simulink model "openloop_SPWM_v2_2020a"  (R2020a)
settings: Solver=ode23tb  StartTime=0.0  StopTime=2  MaxStep=1e-4  RelTol=1e-7
values from neighbouring files (symbols this model uses):
  J = 0.02    [parameter.mat]
  Lm = 0.3197    [parameter.mat]
  Lr = 0.33003    [parameter.mat]
  Ls = 0.33003    [parameter.mat]
  np = 2    [parameter.mat]
  Rr = 2.178    [parameter.mat]
  Rs = 2.804    [parameter.mat]
  Tr = 0.15152892562    [parameter.mat]
libraries: powerlib x9, powerlib_meascontrol x4
settings Model: Creator=Yeblue  LastModifiedBy=EVA
settings DebuggingCC: SFMachineParentedDataDiag=error

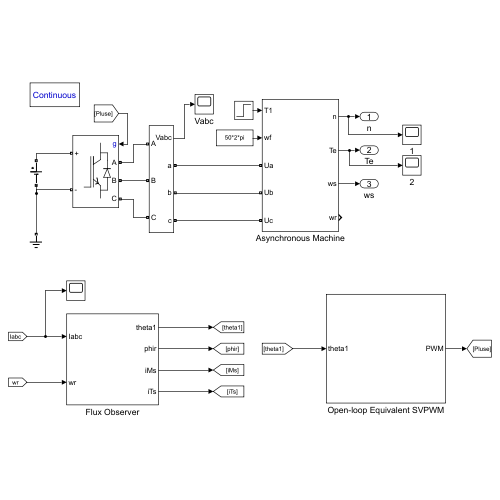
[thumbnail: Simulink's stored preview of the top-level diagram]
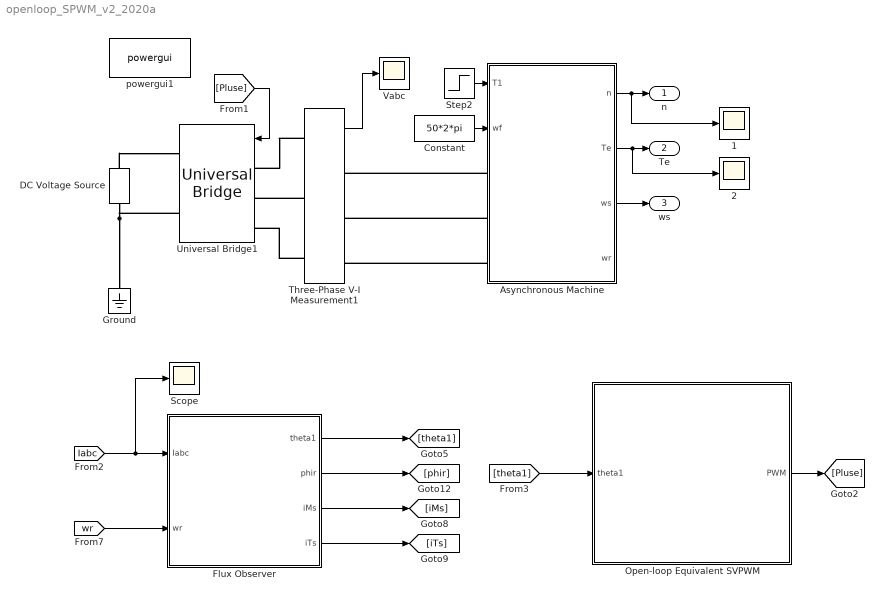
== system openloop_SPWM_v2_2020a ==
  1 : Scope
  2 : Scope
  Asynchronous Machine : Subsystem
  Constant : Constant  Value=50*2*pi
  DC Voltage Source : powerlib/Electrical Sources/DC Voltage Source  Amplitude=380*sqrt(2)/0.5  Measurements=None
  Flux Observer : Subsystem
  Ground : powerlib/Elements/Ground  LConnTagsString=a
  Open-loop Equivalent SVPWM : Subsystem
  Scope : Scope
  Step2 : Step  After=5  SampleTime=0
  Three-Phase V-I Measurement1 : powerlib/Measurements/Three-Phase V-I Measurement  VoltageMeasurement=phase-to-phase  SetLabelV=off  LabelV=Vabc  Vpu=off  VpuLL=off  CurrentMeasurement=no  SetLabelI=off  LabelI=Iabc  Ipu=off  Pbase=100e6  Vbase=500e3  OutputType=Complex  PhasorSimulation=off  PSBequivalent=0
  Universal Bridge1 : powerlib/Power Electronics/Universal Bridge  Arms=3  SnubberResistance=1e5  SnubberCapacitance=inf  Device=IGBT / Diodes  Ron=1e-3  Lon=0  ForwardVoltages="[  0  0  ]"  ForwardVoltage=0  GTOparameters=[ 10e-6 , 20e-6 ]  IGBTparameters=[ 1e-6 , 2e-6 ]  Measurements=None  Measurements_2=None  converterType=Rectifier
  Vabc : Scope
  powergui1 : powerlib/powergui  Priority=1  SimulationMode=Continuous  SampleTime=50e-6  frequency=60  Iterations=50  frequencyindice=0  Pbase=100e6  ErrMax=1e-4  UnitsV=kV  UnitsW=MW  buscounter=0  FunctionMessages=off  echomessages=off  EnableUseOfTLC=off  CurrentSourceSwitches=off  DisableSnubberDevices=off  DisableRonSwitches=off  DisableVfSwitches=off  DisplayEquations=off  AutomaticDiscreteSolvers=off  SolverType=Tustin/Backward Euler (TBE)  Interpol=off  ExternalGateDelay=off  methode=off  Ts=100  x0status=blocks  SPID=on  SwTol=0  HookPort=off  NonlinearTolerance=1e-4  nMaxIteration=100  ContinueOnMaxIteration=off  RestoreLinks=warning  ResistiveCurrentMeasurement=off  Frange=[0:2:500]  Ylog=off  Xlog=on  ShowGrid=off  save=off  variable=ZData  structure=Uab  ZoomFFT=off  StartTime=1.0  cycles=1  DisplayStyle=1  fundamental=50  FreqAxis=on  MaxFrequency=1000  frequencyindicesteady=1  RmsSteady=1  display=off
  n : Outport
  Te : Outport  Port=2
  ws : Outport  Port=3
  wires:
  Asynchronous Machine/2(Te) -> 2/1, Te/1
  Constant/1 -> Asynchronous Machine/2(wf)
  Step2/1 -> Asynchronous Machine/1(T1)
  Flux Observer/2(phir) -> [phir]
  [wr] -> Flux Observer/2(wr)
  [Pluse] -> Universal Bridge1/1
  Flux Observer/4(iTs) -> [iTs]
  Three-Phase V-I Measurement1/1 -> Vabc/1
  Flux Observer/3(iMs) -> [iMs]
  Flux Observer/1(theta1) -> [theta1]
  Asynchronous Machine/1(n) -> n/1, 1/1
  Asynchronous Machine/3(ws) -> ws/1
  [Iabc] -> Scope/1, Flux Observer/1(Iabc)
  Open-loop Equivalent SVPWM/1(PWM) -> [Pluse]
  [theta1] -> Open-loop Equivalent SVPWM/1(theta1)
  connections:
  Universal Bridge1/RConn2 -- Ground/LConn1 -- DC Voltage Source/LConn1
  Asynchronous Machine/LConn2 -- Three-Phase V-I Measurement1/RConn2
  Asynchronous Machine/LConn1 -- Three-Phase V-I Measurement1/RConn1
  Asynchronous Machine/LConn3 -- Three-Phase V-I Measurement1/RConn3
  Three-Phase V-I Measurement1/LConn3 -- Universal Bridge1/LConn3
  Three-Phase V-I Measurement1/LConn1 -- Universal Bridge1/LConn1
  Three-Phase V-I Measurement1/LConn2 -- Universal Bridge1/LConn2
  DC Voltage Source/RConn1 -- Universal Bridge1/RConn1

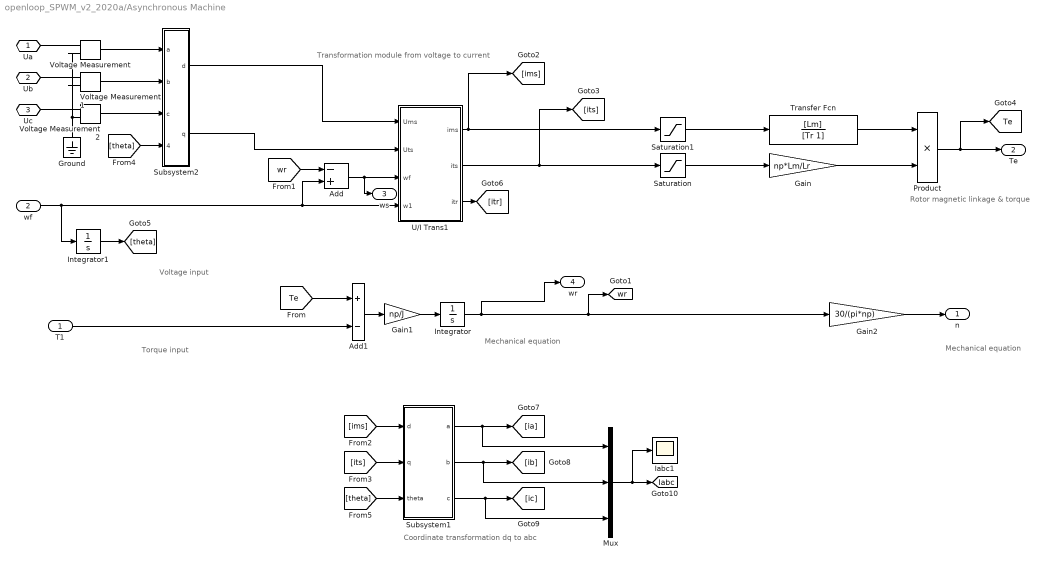
== system openloop_SPWM_v2_2020a/Asynchronous Machine ==
  note: Torque input
  note: Voltage input
  note: Rotor magnetic linkage & torque
  note: Transformation module from voltage to current
  note: Mechanical equation
  note: Coordinate transformation dq to abc
  note: Mechanical equation
  T1 : Inport
  wf : Inport  Port=2
  Add : Sum  Inputs=-+
  Add1 : Sum  Inputs=+-
  Gain : Gain  Gain=np*Lm/Lr
  Gain1 : Gain  Gain=np/J
  Gain2 : Gain  Gain=30/(pi*np)
  Ground : powerlib/Elements/Ground  LConnTagsString=a
  Iabc1 : Scope
  Integrator : Integrator
  Integrator1 : Integrator
  Mux : Mux  Inputs=3
  Product : Product
  Saturation : Saturate  UpperLimit=50  LowerLimit=-50
  Saturation1 : Saturate  UpperLimit=50  LowerLimit=-50
  Subsystem1 : Subsystem
  Subsystem2 : Subsystem
  Transfer Fcn : TransferFcn  Numerator=[Lm]  Denominator=[Tr 1]
  U/I Trans1 : Subsystem
  Voltage Measurement : powerlib/Measurements/Voltage Measurement  PhasorSimulation=off  OutputType=Complex  PSBequivalent=0
  Voltage Measurement1 : powerlib/Measurements/Voltage Measurement  PhasorSimulation=off  OutputType=Complex  PSBequivalent=0
  Voltage Measurement2 : powerlib/Measurements/Voltage Measurement  PhasorSimulation=off  OutputType=Complex  PSBequivalent=0
  Ua : PMIOPort  Side=Left
  Ub : PMIOPort  Port=2  Side=Left
  Uc : PMIOPort  Port=3  Side=Left
  n : Outport
  Te : Outport  Port=2
  ws : Outport  Port=3
  wr : Outport  Port=4
  tag scope: Iabc=global, Te=global, wr=global
  wires:
  Subsystem1/3(c) -> Mux/3, [ic]
  wf/1 -> Integrator1/1, U/I Trans1/4(w1), Add/2
  Product/1 -> Te/1, [Te]
  U/I Trans1/2(its) -> Saturation/1, [its]
  Voltage Measurement2/1 -> Subsystem2/3(c)
  [theta] -> Subsystem2/4(theta)
  Gain2/1 -> n/1
  Add/1 -> ws/1, U/I Trans1/3(wf)
  U/I Trans1/1(ims) -> Saturation1/1, [ims]
  Add1/1 -> Gain1/1
  [theta] -> Subsystem1/3(theta)
  Voltage Measurement1/1 -> Subsystem2/2(b)
  Subsystem2/1(d) -> U/I Trans1/1(Ums)
  [its] -> Subsystem1/2(q)
  Voltage Measurement/1 -> Subsystem2/1(a)
  T1/1 -> Add1/2
  U/I Trans1/3(itr) -> [itr]
  [ims] -> Subsystem1/1(d)
  Integrator1/1 -> [theta]
  Integrator/1 -> [wr], Gain2/1, wr/1
  [wr] -> Add/1
  Gain1/1 -> Integrator/1
  Gain/1 -> Product/2
  Subsystem2/2(q) -> U/I Trans1/2(Uts)
  [Te] -> Add1/1
  Subsystem1/1(a) -> Mux/1, [ia]
  Subsystem1/2(b) -> Mux/2, [ib]
  Transfer Fcn/1 -> Product/1
  Mux/1 -> Iabc1/1, [Iabc]
  Saturation/1 -> Gain/1
  Saturation1/1 -> Transfer Fcn/1
  connections:
  Ground/LConn1 -- Voltage Measurement1/LConn2 -- Voltage Measurement/LConn2 -- Voltage Measurement2/LConn2
  Uc/RConn1 -- Voltage Measurement2/LConn1
  Ub/RConn1 -- Voltage Measurement1/LConn1
  Ua/RConn1 -- Voltage Measurement/LConn1

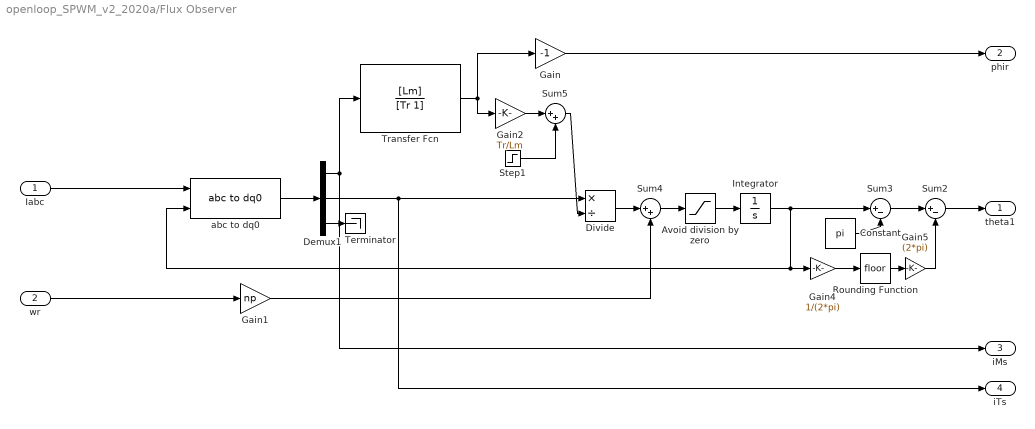
== system openloop_SPWM_v2_2020a/Flux Observer ==
  Iabc : Inport
  wr : Inport  Port=2
  Avoid division by zero : Saturate  UpperLimit=1e6  LowerLimit=1e-6
  Constant : Constant  Value=pi
  Demux1 : Demux  Outputs=3
  Divide : Product  Inputs=*/
  Gain : Gain  Gain=-1
  Gain1 : Gain  Gain=np
  Gain2 : Gain  Gain=Tr/Lm
  Gain4 : Gain  Gain=1/(2*pi)
  Gain5 : Gain  Gain=(2*pi)
  Integrator : Integrator  InitialCondition=10.00001
  Rounding Function : Rounding
  Step1 : Step  Time=0.01  Before=1000  After=0  SampleTime=0
  Sum2 : Sum  Inputs=|+-
  Sum3 : Sum  Inputs=|+-
  Sum4 : Sum  Inputs=|++
  Sum5 : Sum  Inputs=|++
  Terminator : Terminator
  Transfer Fcn : TransferFcn  Numerator=[Lm]  Denominator=[Tr 1]
  abc to dq0 : powerlib_meascontrol/Transformations/abc to dq0  Alignment=90 degrees behind phase A axis
  theta1 : Outport  VectorParamsAs1DForOutWhenUnconnected=off
  phir : Outport  Port=2  VectorParamsAs1DForOutWhenUnconnected=off
  iMs : Outport  Port=3  VectorParamsAs1DForOutWhenUnconnected=off
  iTs : Outport  Port=4  VectorParamsAs1DForOutWhenUnconnected=off
  wires:
  Divide/1 -> Sum4/1
  Step1/1 -> Sum5/2
  Sum5/1 -> Divide/2
  wr/1 -> Gain1/1
  Gain2/1 -> Sum5/1
  abc to dq0/1 -> Demux1/1
  Transfer Fcn/1 -> Gain/1, Gain2/1
  Iabc/1 -> abc to dq0/1
  Demux1/3 -> Terminator/1
  Demux1/1 -> iMs/1, Transfer Fcn/1
  Demux1/2 -> iTs/1, Divide/1
  Sum3/1 -> Sum2/1
  Sum2/1 -> theta1/1
  Constant/1 -> Sum3/2
  Rounding Function/1 -> Gain5/1
  Gain5/1 -> Sum2/2
  Gain4/1 -> Rounding Function/1
  Gain1/1 -> Sum4/2
  Gain/1 -> phir/1
  Sum4/1 -> Avoid division by zero/1
  Integrator/1 -> Sum3/1, Gain4/1, abc to dq0/2
  Avoid division by zero/1 -> Integrator/1

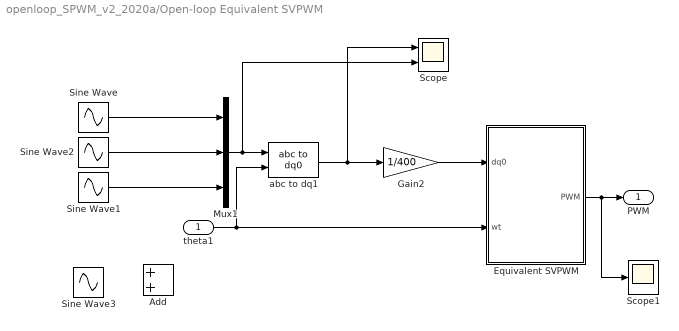
== system openloop_SPWM_v2_2020a/Open-loop Equivalent SVPWM ==
  theta1 : Inport
  Add : Sum
  Equivalent SVPWM : Subsystem
  Gain2 : Gain  Gain=1/400
  Mux1 : Mux  Inputs=3
  Scope : Scope  NumInputPorts=2
  Scope1 : Scope
  Sine Wave : Sin  Amplitude=380  Frequency=314.16  SampleTime=0
  Sine Wave1 : Sin  Amplitude=380  Frequency=314.16  Phase=2.0944  SampleTime=0
  Sine Wave2 : Sin  Amplitude=380  Frequency=314.16  Phase=4.1888  SampleTime=0
  Sine Wave3 : Sin  Amplitude=63.3333  Frequency=942.48  SampleTime=0
  abc to dq1 : powerlib_meascontrol/Transformations/abc to dq0  Alignment=90 degrees behind phase A axis
  PWM : Outport  VectorParamsAs1DForOutWhenUnconnected=off
  wires:
  theta1/1 -> Equivalent SVPWM/2(wt), abc to dq1/2
  Gain2/1 -> Equivalent SVPWM/1(dq0)
  Equivalent SVPWM/1(PWM) -> Scope1/1, PWM/1
  Sine Wave2/1 -> Mux1/2
  Sine Wave/1 -> Mux1/1
  Mux1/1 -> Scope/2, abc to dq1/1
  abc to dq1/1 -> Scope/1, Gain2/1
  Sine Wave1/1 -> Mux1/3

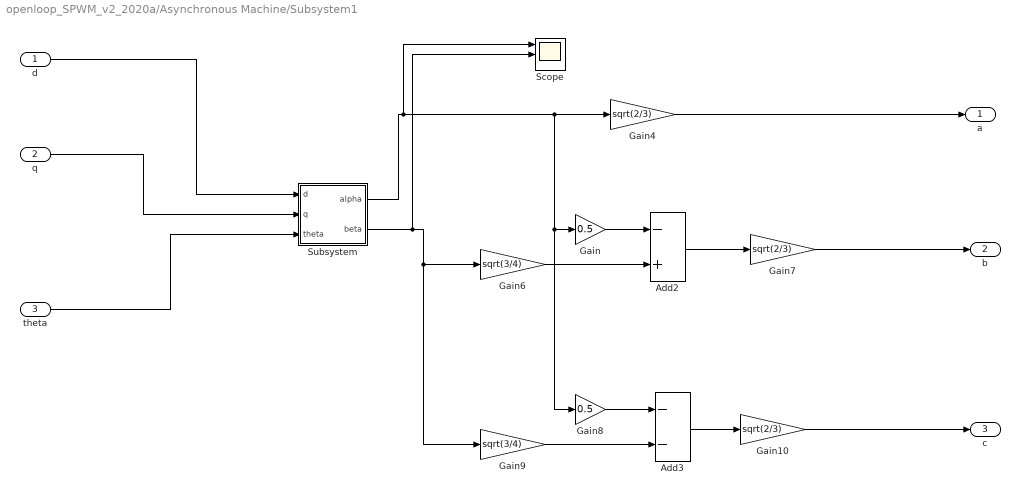
== system openloop_SPWM_v2_2020a/Asynchronous Machine/Subsystem1 ==
  d : Inport
  q : Inport  Port=2
  theta : Inport  Port=3
  Add2 : Sum  Inputs=-+
  Add3 : Sum  Inputs=--
  Gain : Gain  Gain=0.5
  Gain10 : Gain  Gain=sqrt(2/3)
  Gain4 : Gain  Gain=sqrt(2/3)
  Gain6 : Gain  Gain=sqrt(3/4)
  Gain7 : Gain  Gain=sqrt(2/3)
  Gain8 : Gain  Gain=0.5
  Gain9 : Gain  Gain=sqrt(3/4)
  Scope : Scope  NumInputPorts=3
  Subsystem : Subsystem
  a : Outport
  b : Outport  Port=2
  c : Outport  Port=3
  wires:
  Gain10/1 -> c/1
  Gain4/1 -> a/1
  Subsystem/2(beta) -> Scope/2, Gain9/1, Gain6/1
  q/1 -> Subsystem/2(q)
  theta/1 -> Subsystem/3(theta)
  d/1 -> Subsystem/1(d)
  Gain6/1 -> Add2/2
  Subsystem/1(alpha) -> Scope/1, Gain8/1, Gain/1, Gain4/1
  Add2/1 -> Gain7/1
  Gain9/1 -> Add3/2
  Gain7/1 -> b/1
  Add3/1 -> Gain10/1
  Gain/1 -> Add2/1
  Gain8/1 -> Add3/1

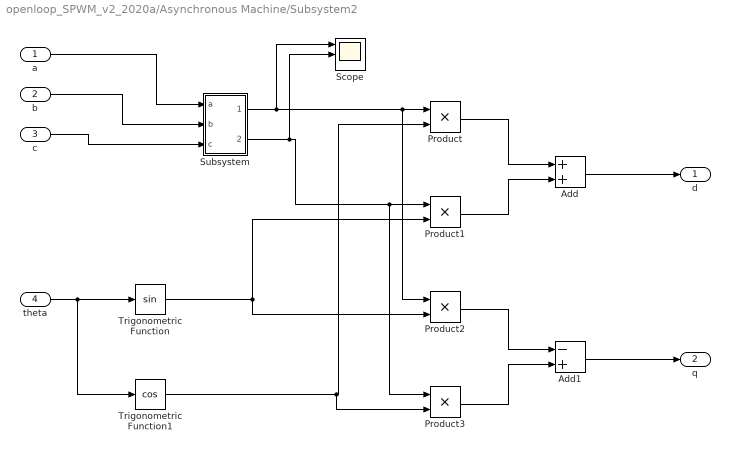
== system openloop_SPWM_v2_2020a/Asynchronous Machine/Subsystem2 ==
  a : Inport
  b : Inport  Port=2
  c : Inport  Port=3
  theta : Inport  Port=4
  Add : Sum
  Add1 : Sum  Inputs=-+
  Product{,1..3} (4 alike) : Product
  Scope : Scope  NumInputPorts=3
  Subsystem : Subsystem
  Trigonometric Function : Trigonometry
  Trigonometric Function1 : Trigonometry  Operator=cos
  d : Outport
  q : Outport  Port=2
  wires:
  Trigonometric Function1/1 -> Product3/2, Product/2
  Trigonometric Function/1 -> Product2/2, Product1/2
  Product/1 -> Add/1
  c/1 -> Subsystem/3(c)
  Subsystem/2(beta) -> Scope/2, Product3/1, Product1/1
  a/1 -> Subsystem/1(a)
  Product1/1 -> Add/2
  b/1 -> Subsystem/2(b)
  Subsystem/1(alpha) -> Scope/1, Product2/1, Product/1
  Product3/1 -> Add1/2
  theta/1 -> Trigonometric Function1/1, Trigonometric Function/1
  Product2/1 -> Add1/1
  Add1/1 -> q/1
  Add/1 -> d/1

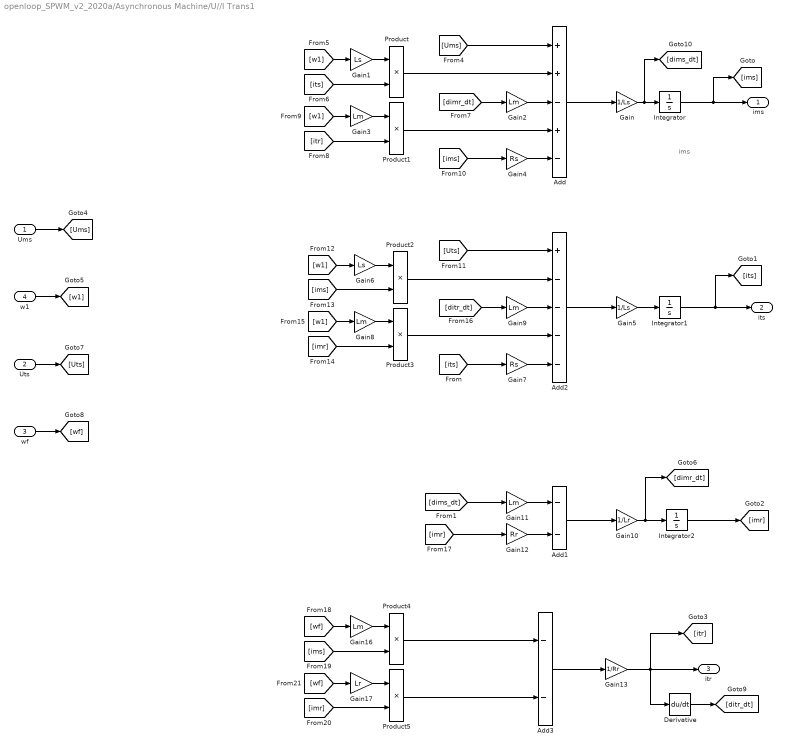
== system openloop_SPWM_v2_2020a/Asynchronous Machine/U//I Trans1 ==
  note: ims
  Ums : Inport
  Uts : Inport  Port=2
  wf : Inport  Port=3
  w1 : Inport  Port=4
  Add : Sum  Inputs=++-+-
  Add1 : Sum  Inputs=--
  Add2 : Sum  Inputs=+----
  Add3 : Sum  Inputs=--
  Derivative : Derivative
  Gain : Gain  Gain=1/Ls
  Gain1 : Gain  Gain=Ls
  Gain10 : Gain  Gain=1/Lr
  Gain{2..3,8..9,11,16} (6 alike) : Gain  Gain=Lm
  Gain12 : Gain  Gain=Rr
  Gain13 : Gain  Gain=1/Rr
  Gain17 : Gain  Gain=Lr
  Gain4 : Gain  Gain=Rs
  Gain5 : Gain  Gain=1/Ls
  Gain6 : Gain  Gain=Ls
  Gain7 : Gain  Gain=Rs
  Integrator : Integrator
  Integrator1 : Integrator
  Integrator2 : Integrator
  Product{,1..5} (6 alike) : Product
  ims : Outport
  its : Outport  Port=2
  itr : Outport  Port=3
  wires:
  Gain6/1 -> Product2/1
  [dimr_dt] -> Gain2/1
  Gain/1 -> Integrator/1, [dims_dt]
  Product2/1 -> Add2/2
  Gain8/1 -> Product3/1
  Add/1 -> Gain/1
  w1/1 -> [w1]
  Gain10/1 -> [dimr_dt], Integrator2/1
  wf/1 -> [wf]
  Integrator/1 -> ims/1, [ims]
  [dims_dt] -> Gain11/1
  [ims] -> Product4/2
  Gain9/1 -> Add2/3
  [imr] -> Product3/2
  [itr] -> Product1/2
  Gain2/1 -> Add/3
  [w1] -> Gain8/1
  [wf] -> Gain16/1
  Product3/1 -> Add2/4
  Integrator1/1 -> its/1, [its]
  Gain13/1 -> itr/1, Derivative/1, [itr]
  [w1] -> Gain3/1
  Gain16/1 -> Product4/1
  Gain5/1 -> Integrator1/1
  [Ums] -> Add/1
  [Uts] -> Add2/1
  Integrator2/1 -> [imr]
  Product4/1 -> Add3/1
  [its] -> Gain7/1
  Product1/1 -> Add/4
  Ums/1 -> [Ums]
  [imr] -> Product5/2
  Gain1/1 -> Product/1
  [ims] -> Product2/2
  [w1] -> Gain6/1
  [wf] -> Gain17/1
  [imr] -> Gain12/1
  Product/1 -> Add/2
  Gain11/1 -> Add1/1
  Uts/1 -> [Uts]
  Gain4/1 -> Add/5
  [ims] -> Gain4/1
  Gain7/1 -> Add2/5
  Add1/1 -> Gain10/1
  [its] -> Product/2
  Derivative/1 -> [ditr_dt]
  Add2/1 -> Gain5/1
  Product5/1 -> Add3/2
  Gain17/1 -> Product5/1
  Gain3/1 -> Product1/1
  [ditr_dt] -> Gain9/1
  [w1] -> Gain1/1
  Gain12/1 -> Add1/2
  Add3/1 -> Gain13/1

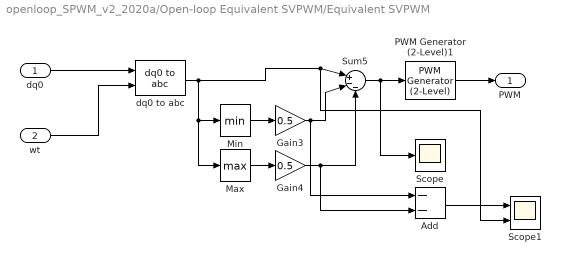
== system openloop_SPWM_v2_2020a/Open-loop Equivalent SVPWM/Equivalent SVPWM ==
  dq0 : Inport
  wt : Inport  Port=2
  Add : Sum  Inputs=--
  Gain3 : Gain  Gain=0.5
  Gain4 : Gain  Gain=0.5
  Max : MinMax  Function=max
  Min : MinMax
  PWM Generator (2-Level)1 : powerlib_meascontrol/Pulse & Signal Generators/PWM Generator (2-Level)  ModulatorType=Three-phase bridge (6 pulses)  ModulatorMode=Unsynchronized  Fc=20e3  Pc=90  nF=27  MinMax="[ -1  1 ]"  SamplingTechnique=Symmetrical regular (single edge)  ModulatingSignals=off  m=0.8  Freq=60  Phase=0  Ts=0  ShowCarrierOutport=off
  Scope : Scope
  Scope1 : Scope  NumInputPorts=2
  Sum5 : Sum  Inputs=|+--
  dq0 to abc : powerlib_meascontrol/Transformations/dq0 to abc  Alignment=90 degrees behind phase A axis
  PWM : Outport  VectorParamsAs1DForOutWhenUnconnected=off
  wires:
  wt/1 -> dq0 to abc/2
  Min/1 -> Gain3/1
  Gain4/1 -> Add/2, Sum5/3
  Max/1 -> Gain4/1
  Gain3/1 -> Add/1, Sum5/2
  dq0 to abc/1 -> Max/1, Min/1, Scope1/2, Sum5/1
  Sum5/1 -> Scope/1, PWM Generator (2-Level)1/1
  dq0/1 -> dq0 to abc/1
  PWM Generator (2-Level)1/1 -> PWM/1
  Add/1 -> Scope1/1

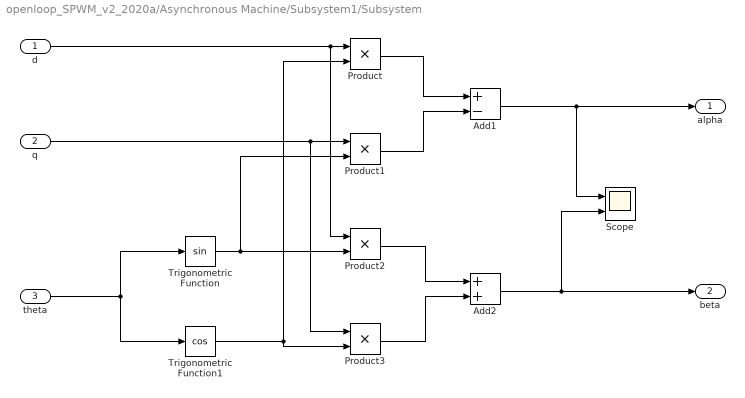
== system openloop_SPWM_v2_2020a/Asynchronous Machine/Subsystem1/Subsystem ==
  d : Inport
  q : Inport  Port=2
  theta : Inport  Port=3
  Add1 : Sum  Inputs=+-
  Add2 : Sum
  Product{,1..3} (4 alike) : Product
  Scope : Scope  NumInputPorts=2
  Trigonometric Function : Trigonometry
  Trigonometric Function1 : Trigonometry  Operator=cos
  alpha : Outport
  beta : Outport  Port=2
  wires:
  Product/1 -> Add1/1
  Add1/1 -> Scope/1, alpha/1
  q/1 -> Product3/1, Product1/1
  Product2/1 -> Add2/1
  Product1/1 -> Add1/2
  Trigonometric Function/1 -> Product2/2, Product1/2
  Product3/1 -> Add2/2
  Add2/1 -> Scope/2, beta/1
  d/1 -> Product2/1, Product/1
  theta/1 -> Trigonometric Function/1, Trigonometric Function1/1
  Trigonometric Function1/1 -> Product/2, Product3/2

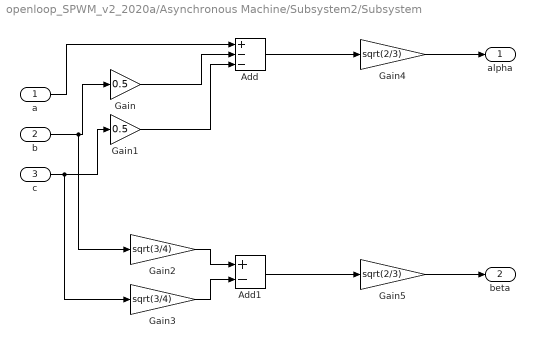
== system openloop_SPWM_v2_2020a/Asynchronous Machine/Subsystem2/Subsystem ==
  a : Inport
  b : Inport  Port=2
  c : Inport  Port=3
  Add : Sum  Inputs=+--
  Add1 : Sum  Inputs=+-
  Gain : Gain  Gain=0.5
  Gain1 : Gain  Gain=0.5
  Gain2 : Gain  Gain=sqrt(3/4)
  Gain3 : Gain  Gain=sqrt(3/4)
  Gain4 : Gain  Gain=sqrt(2/3)
  Gain5 : Gain  Gain=sqrt(2/3)
  alpha : Outport
  beta : Outport  Port=2
  wires:
  Add/1 -> Gain4/1
  b/1 -> Gain2/1, Gain/1
  Gain2/1 -> Add1/1
  Gain4/1 -> alpha/1
  Add1/1 -> Gain5/1
  c/1 -> Gain3/1, Gain1/1
  Gain/1 -> Add/2
  Gain3/1 -> Add1/2
  Gain5/1 -> beta/1
  a/1 -> Add/1
  Gain1/1 -> Add/3
